simulink model "goto_1"  (Simulink 4.00)
settings: Solver=ode45  StartTime=0.0  StopTime=10.0  RelTol=1e-3
libraries: simulink3 x1
settings Model: LastModifiedBy=Administrator  BlockReductionOpt=off

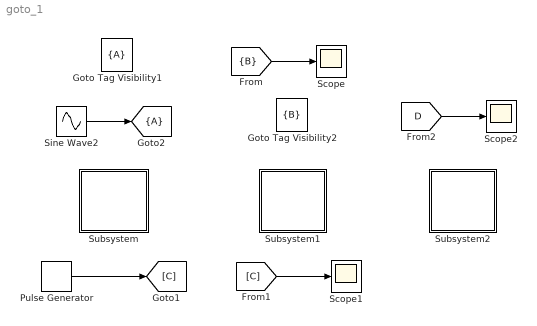
== system goto_1 ==
  Goto Tag Visibility1 : GotoTagVisibility  GotoTag=A
  Goto Tag Visibility2 : GotoTagVisibility  GotoTag=B
  Pulse Generator : simulink3/Sources/Pulse Generator  period=1  duty=50  amplitude=1  start=0
  Scope : Scope
      settings: TimeRange=auto  YMin=-5  YMax=5  SaveToWorkspace=off  LimitDataPoints=on  MaxDataPoints=5000
  Scope1 : Scope
      settings: TimeRange=auto  YMin=-5  YMax=5  SaveToWorkspace=off  SaveName=ScopeData2  LimitDataPoints=on  MaxDataPoints=5000
  Scope2 : Scope
      settings: TimeRange=auto  YMin=-5  YMax=5  SaveToWorkspace=off  SaveName=ScopeData3  LimitDataPoints=on  MaxDataPoints=5000
  Sine Wave2 : Sin  Amplitude=1  Frequency=1  Phase=0  SampleTime=0
  Subsystem : Subsystem
      settings: RTWFcnNameOpts=Auto  RTWFileNameOpts=Auto
  Subsystem1 : Subsystem
      settings: RTWFcnNameOpts=Auto  RTWFileNameOpts=Auto
  Subsystem2 : Subsystem
      settings: RTWFcnNameOpts=Auto  RTWFileNameOpts=Auto
  tag scope: A=scoped
  wires:
  [B] -> Scope/1
  Sine Wave2/1 -> [A]
  [C] -> Scope1/1
  Pulse Generator/1 -> [C]
  [D] -> Scope2/1

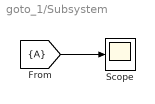
== system goto_1/Subsystem ==
  Scope : Scope
      settings: TimeRange=auto  YMin=-5  YMax=5  SaveToWorkspace=off  SaveName=ScopeData  LimitDataPoints=on  MaxDataPoints=5000
  wires:
  [A] -> Scope/1

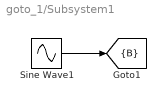
== system goto_1/Subsystem1 ==
  Sine Wave1 : Sin  Amplitude=1  Frequency=4  Phase=0  SampleTime=0
  tag scope: B=scoped
  wires:
  Sine Wave1/1 -> [B]

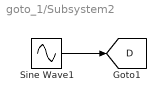
== system goto_1/Subsystem2 ==
  Sine Wave1 : Sin  Amplitude=1  Frequency=4  Phase=0  SampleTime=0
  tag scope: D=global
  wires:
  Sine Wave1/1 -> [D]
